simulink model "Lab1PartA1"  (R2023a)
settings: Solver=VariableStepAuto  StartTime=0.0  StopTime=20  RelTol=1e-3
settings Model: Creator=m96sz  LastModifiedBy=m96sz

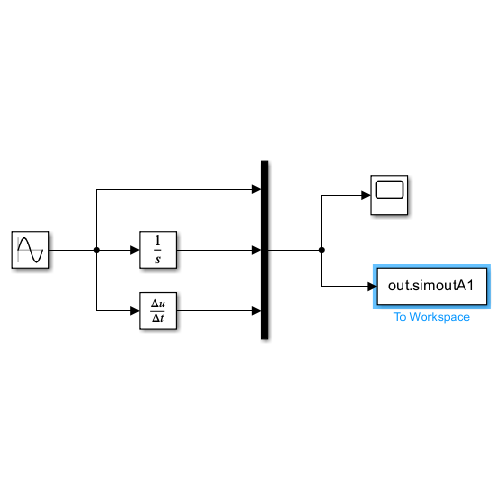
[thumbnail: Simulink's stored preview of the top-level diagram]
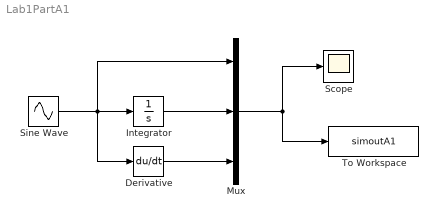
== system Lab1PartA1 ==
  Derivative : Derivative
  Integrator : Integrator
  Mux : Mux  Inputs=3
  Scope : Scope
  Sine Wave : Sin  Frequency=1.257  SampleTime=0
  To Workspace : ToWorkspace  VariableName=simoutA1  SampleTime=-1
  wires:
  Mux/1 -> Scope/1, To Workspace/1
  Sine Wave/1 -> Mux/1, Derivative/1, Integrator/1
  Integrator/1 -> Mux/2
  Derivative/1 -> Mux/3
